simulink library "Scissor_Parts_Lib"  (R2017a)
settings: Solver=ode45  StartTime=0.0  StopTime=10.0  RelTol=1e-3  EnableMultiTasking=on
undefined symbols (not defined in the file): Blue, Extr_Data_LinkHoles, Extr_Data_Ring, Gray, Local, Scissor_Lift_Param, X, Y, Z
libraries: sm_lib x52, Scissor_Parts_Lib x16
(part 1 of 2)
Description:
  | Copyright 2014-2017 The MathWorks, Inc.
settings Model: Creator=smiller  LastModifiedBy=smiller
settings DataIOCC: LimitDataPoints=on  SaveFormat=Array  SignalLoggingSaveFormat=ModelDataLogs
settings OptimizationCC: ExpressionDepthLimit=2147483647  LifeSpan=inf
settings DebuggingCC: UnderspecifiedInitializationDetection=Classic  MergeDetectMultiDrivingBlocksExec=none  SolverPrmCheckMsg=warning  FcnCallInpInsideContextMsg=warning  AllowSymbolicDim=off  StateNameClashWarn=warning  SFUnexpectedBacktrackingDiag=warning  SFNoUnconditionalDefaultTransitionDiag=warning  SFExecutionAtInitializationDiag=none
settings HardwareCC: ProdBitPerPointer=32  ProdBitPerSizeT=32  ProdBitPerPtrDiffT=32  ProdLargestAtomicFloat=None  ProdIntDivRoundTo=Undefined  ProdEndianess=Unspecified  ProdWordSize=32  ProdHWDeviceType=32-bit Generic
settings ModelReferenceCC: PropagateSignalLabelsOutOfModel=off
settings GRTTargetCC: TargetLangStandard=C89/C90 (ANSI)  GeneratePreprocessorConditionals=Disable all
settings ConfigComp: CovMetricSettings=dw  CovHtmlReporting=on  CovSaveCumulativeToWorkspaceVar=on  CovSaveSingleToWorkspaceVar=on  CovExternalEMLEnable=off  CovSFcnEnable=off

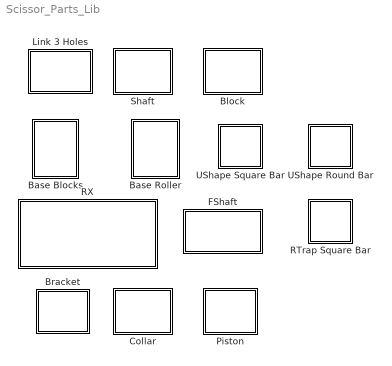
== system Scissor_Parts_Lib ==
  Base Blocks : Subsystem  mask(Base Blocks){block_length=Scissor_Lift_Param.Base_Block.Length, block_width=Scissor_Lift_Param.Base_Block.Width, block_height=Scissor_Lift_Param.Base_Block.Height, shaft_radius=Scissor_Lift_Param.Roller.Shaft_Radius, shaft_length=Scissor_Lift_Param.Roller.Shaft_Length, material_density=Scissor_Lift_Param.Base_Block.Density, material_color=Scissor_Lift_Param.Base_Block.Color, material_opacity=Scissor_Lift_Param.Base_Block.Opacity}
      mask prompts: block_length "Length (cm)"; block_width "Width (cm)"; block_height "Height (cm)"; shaft_radius "Radius (cm)"; shaft_length "Length (cm)"; material_density "Density (kg/m^3)"; material_color "Color"; material_opacity "Opacity"
      mask help: Parameterized base with two blocks and a shaft.
      mask Display:
      | image(imread('Base_Blocks_IMAGE.jpg'));
      | port_label('RConn',1,'S');
      | port_label('LConn',1,'B');
  Base Roller : Subsystem  mask(Base Roller){roller_length=Scissor_Lift_Param.Roller.Roller_Length, roller_radius=Scissor_Lift_Param.Roller.Roller_Radius, shaft_length=Scissor_Lift_Param.Roller.Shaft_Length, shaft_radius=Scissor_Lift_Param.Roller.Shaft_Radius, material_density=Scissor_Lift_Param.Roller.Density, material_color=Scissor_Lift_Param.Roller.Color, material_opacity=Scissor_Lift_Param.Roller.Opacity}
      mask prompts: roller_length "Length (cm)"; roller_radius "Radius (cm)"; shaft_length "Length (cm)"; shaft_radius "Radius (cm)"; material_density "Density (kg/m^3)"; material_color "Color"; material_opacity "Opacity"
      mask help: Parameterized roller with two wheels connected by a shaft.
      mask Display:
      | image(imread('Base_Roller_IMAGE.jpg'));
      | port_label('RConn',1,'S');
      | port_label('LConn',1,'B');
  Block : Subsystem  mask(Block){L=Scissor_Lift_Param.Base_Block.Length, W=Scissor_Lift_Param.Base_Block.Width, H=Scissor_Lift_Param.Base_Block.Height, z_ori=Local +Z, rho=Scissor_Lift_Param.Base_Block.Density, clr=Scissor_Lift_Param.Base_Block.Color, opc=Scissor_Lift_Param.Base_Block.Opacity}
      mask prompts: L "Length (cm):"; W "Width (cm):"; H "Height (cm):"; z_ori "Shaft orientation:"; rho "Shaft density (kg/m^3):"; clr "Link color:"; opc "Opacity:"
      mask help: Rectangular block. Ports are at the center of the faces normal to the local z-axis. Can be configured to have positive Z from B to F or from F to B.
      mask init:
      | if(z_ori == 2)
      |     z_ori = -1;
      | end
      mask TypeOptions z_ori: Local +Z | Local -Z
      mask Display:
      | image(imread('Block_IMAGE.jpg'));
      | port_label('LConn',1,'B');
      | port_label('RConn',1,'F');
  Bracket : Subsystem  mask(Actuation Bracket){fl_w=Scissor_Lift_Param.Actuator.Bracket.Flange.Width, fl_h=Scissor_Lift_Param.Actuator.Bracket.Flange.Height, T=Scissor_Lift_Param.Actuator.Bracket.Flange.Thickness, W=Scissor_Lift_Param.Actuator.Bracket.Flange.Offset, flupdown=Down, flfrontrear=Rear, fl_density=Scissor_Lift_Param.Actuator.Bracket.Flange.Density, fl_clr=Scissor_Lift_Param.Actuator.Bracket.Flange.Color, fl_opc=Scissor_Lift_Param.Actuator.Bracket.Flange.Opacity, shaft_length=Scissor_Lift_Param.Link_Separation.Outer_Outer-Scissor_Lift_Param.Link_Separation.Outer_Inner*2, shaft_radius=Scissor_Lift_Param.Actuator.Bracket.Shaft.Radius, shaft_density=Scissor_Lift_Param.Actuator.Bracket.Shaft.Density, shaft_color=Scissor_Lift_Param.Actuator.Bracket.Shaft.Color, shaft_opacity=Scissor_Lift_Param.Actuator.Bracket.Shaft.Opacity}
      mask prompts: fl_w "Width (cm)"; fl_h "Height (cm)"; T "Thickness (cm)"; W "Offset (cm)"; flupdown "Orientation"; flfrontrear "Position"; fl_density "Density"; fl_clr "Color"; fl_opc "Opacity"; shaft_length "Length (cm)"; shaft_radius "Radius (cm)"; shaft_density "Density (kg/m^3)"; shaft_color "Color"; shaft_opacity "Opacity"
      mask help: Actuation bracket for scissor lift mechanism. Contains flanges that attach to links and connection shaft. Configurable orientation and surface attachment.
      mask init:
      | if(flupdown == 2)
      |     flupdown = -1;
      | end
      | if(flfrontrear == 2)
      |     flfrontrear = -1;
      | end
      mask TypeOptions flupdown: Down | Up
      mask TypeOptions flfrontrear: Front | Rear
      mask Display:
      | image(imread('Bracket_IMAGE.jpg'));
      | port_label('RConn',1,'F');
      | port_label('RConn',2,'B');
      | port_label('LConn',1,'C');
  Collar : Subsystem  mask{collar_length=Scissor_Lift_Param.Actuator.Collar.Length, collar_radius=Scissor_Lift_Param.Actuator.Collar.Radius, cylinder_length=Scissor_Lift_Param.Actuator.Piston_Seat.Length, cylinder_radius=Scissor_Lift_Param.Actuator.Piston_Seat.Radius, cylinder_ori=Local +Z, material_density=Scissor_Lift_Param.Actuator.Collar.Density, material_color=Scissor_Lift_Param.Actuator.Collar.Color, material_opacity=Scissor_Lift_Param.Actuator.Collar.Opacity}
      mask prompts: collar_length "Length (cm):"; collar_radius "Radius (cm):"; cylinder_length "Length (cm):"; cylinder_radius "Radius (cm):"; cylinder_ori "Orientation (B to C):"; material_density "Density (kg/m^3):"; material_color "Color:"; material_opacity "Opacity:"
      mask init:
      | if(cylinder_ori == 2)
      |     cylinder_ori = -1;
      | end
      mask TypeOptions cylinder_ori: Local +Z | Local -Z
      mask Display:
      | image(imread('Actuator_Collar_IMAGE.jpg'));
      | port_label('LConn',1,'B');
      | port_label('RConn',1,'C');
  FShaft : Subsystem  mask(Transverse Shaft){sep_outer_outer=Scissor_Lift_Param.Link_Separation.Outer_Outer, sep_outer_inner=Scissor_Lift_Param.Link_Separation.Outer_Inner, shaft_radius=Scissor_Lift_Param.Trans_Shaft.Radius, shaft_density=Scissor_Lift_Param.Trans_Shaft.Density, shaft_color=Scissor_Lift_Param.Trans_Shaft.Color, shaft_opacity=Scissor_Lift_Param.Trans_Shaft.Opacity}
      mask prompts: sep_outer_outer "Outer connection separation (cm)"; sep_outer_inner "Outer to inner separation (cm)"; shaft_radius "Radius (cm)"; shaft_density "Density (kg/m^3)"; shaft_color "Color"; shaft_opacity "Opacity"
      mask help: Transverse shaft with four connections. Frames are located at shaft center, with Z-axis along center.
      mask Display:
      | image(imread('Shaft_IMAGE.jpg'));
      | port_label('LConn',1,'LO');
      | port_label('LConn',2,'LI');
      | port_label('RConn',1,'RO');
      | port_label('RConn',2,'RI');
  Link 3 Holes : Subsystem  mask(Connector Link, 3 Holes){L=240, W=15, T=4, r=5, rho=1000, clr_string=Gray, opc=1}
      mask prompts: L "Link length (cm):"; W "Link width (cm):"; T "Link thickness (cm):"; r "Hole radius (cm):"; rho "Density (kg/m^3):"; clr_string "Color:"; opc "Opacity:"
      mask help: Connector link with holes. Ports are located at centers of holes, oriented such that Z is out of the hole, positive X is from L hole to R hole.
      mask init:
      | imgfile='Link_3_Hole_Yellow_IMAGE.jpg';
      | if(strcmp(clr_string,'Yellow'))
      |     clr = [0.6 0.6 0.0];
      | elseif(strcmp(clr_string,'Red'))
      |     clr = [0.8 0.2 0.0];
      |     imgfile='Link_3_Hole_Red_IMAGE.jpg';
      | elseif(strcmp(clr_string,'Gray'))
      |     clr = [0.9 0.9 0.9];
      |     imgfile='Link_3_Hole_Gray_IMAGE.jpg';
      | elseif(strcmp(clr_string,'Gray-Blue'))
      |     clr = [164 184 200]/255;
      |     imgfile='Link_3_Hole_GrayBlue_IMAGE.jpg';
      | end
      mask TypeOptions clr_string: Yellow | Red | Gray | Gray-Blue
      mask Display:
      | image(imread(imgfile));
      | port_label('RConn',1,'F');
      | port_label('RConn',2,'C');
      | port_label('RConn',3,'R');
  Piston : Subsystem
      mask Display:
      | image(imread('Piston_Shaft_IMAGE.jpg'));
      | port_label('RConn',1,'P');
      | port_label('LConn',1,'R');
  RTrap Square Bar : Subsystem  mask(U-Shape from Round Bar){pipe_width=5, height_c1=30, height_c2=60, rail_curve_rad1=20, rail_curve_rad2=20, curve_ang1=60, curve_ang2=45, width=150, clr=[0 0.6 0.8], rho=0.01}
      mask prompts: pipe_width "Pipe Width (cm)"; width "Width (cm)"; clr "Color"; rho "Density"
      mask help: U-Shape formed from a bar with square cross-section
      mask DialogControl Control2 Prompt: Curve 1
      mask DialogControl Control3 Prompt: Curve 2
      mask DialogControl Control7 Prompt: Height (cm)
      mask DialogControl Control8 Prompt: Curve Radius (cm)
      mask DialogControl Control9 Prompt: Angle (deg)
  RX : Subsystem  mask(Scissor Lift Crossbar){link_length=Scissor_Lift_Param.Link.Length, link_width=Scissor_Lift_Param.Link.Width, link_thickness=Scissor_Lift_Param.Link.Thickness, link_hole_radius=Scissor_Lift_Param.Link.Hole_Radius, link_density=Scissor_Lift_Param.Link.Density, link_color=Scissor_Lift_Param.Link.Color, link_opacity=Scissor_Lift_Param.Link.Opacity, shaft_length=Scissor_Lift_Param.Link_Separation.Outer_Inner, shaft_radius=Scissor_Lift_Param.Link_Pin.Radius, shaft_density=Scissor_Lift_Param.Link_Pin.Density, shaft_color=Scissor_Lift_Param.Link_Pin.Color, shaft_opacity=Scissor_Lift_Param.Link_Pin.Opacity, leftright=Right, imgfile=Crossbar_RX_IMAGE.jpg, L1Port=OU, L2Port=IU, R1Port=OL, R2Port=IL}
      mask prompts: link_length "Length (cm)"; link_width "Width (cm)"; link_thickness "Thickness (cm)"; link_hole_radius "Hole Radius (cm)"; link_density "Density (kg/m^3)"; link_color "Color"; link_opacity "Opacity"; shaft_length "Length (cm)"; shaft_radius "Radius (cm)"; shaft_density "Density (kg/m^3)"; shaft_color "Color"; shaft_opacity "Opacity"; leftright "Side"; imgfile "Image File"; L1Port "L1 Port Name"; L2Port "L2 Port Name"; R1Port "R1 Port Name"; R2Port "R2 Port Name"
      mask help: Parameterized crossbar. The two links are connected by a revolute joint. Configurable for left or right side.
      mask init:
      | pinbpth = find_system(gcb,'LookUnderMasks','on','FollowLinks','on','Regexp','on','BlockDialogParams','^Local');
      | %get_param(pinbpth,'z_ori')
      | %leftright
      | %if(1==2)
      | if (leftright == 1)
      |     %disp('Setting to 0, LEFT');
      |     set_param(char(pinbpth),'z_ori',1);
      |     set_param([gcb '/OL'],'Port','1','Side','Right');
      |     set_param([gcb '/IL'],'Port','2','Side','Right');
      |     set_param([gcb '/OU'],'Port','3','Side','Left');
      |     set_param([gcb '/IU'],'Port','4','Side','Left');
      |     set_param(gcb,'Name','LX');
      |     L1Port='OU';
      |     L2Port='IU';
      |     R1Port='OL';
      |     R2Port='IL';
      |     imgfile = 'Crossbar_LX_IMAGE.jpg';
      | else
      |     %disp('Setting to 1, RIGHT');
      |     set_param(char(pinbpth),'z_ori',0);
      |     set_param([gcb '/IL'],'Port','1','Side','Right');
      |     set_param([gcb '/OL'],'Port','2','Side','Right');
      |     set_param([gcb '/IU'],'Port','3','Side','Left');
      |     set_param([gcb '/OU'],'Port','4','Side','Left');
      |     set_param(gcb,'Name','RX');
      |     L1Port='IU';
      |     L2Port='OU';
      |     R1Port='IL';
      |     R2Port='OL';
      |     imgfile = 'Crossbar_RX_IMAGE.jpg';
      | end
      | %end
      mask TypeOptions leftright: Left | Right
      mask Display:
      | image(imread(imgfile));
      | port_label('LConn',1,L1Port);
      | port_label('LConn',2,L2Port);
      | port_label('RConn',1,R1Port);
      | port_label('RConn',2,R2Port);
  Shaft : Subsystem  mask(Cylindrical Shaft){L=10, r=5, theta=0, z_ori=Local -Z, Ro=1000, clr=[0.0 0.6 0.8], opc=1}
      mask prompts: L "Length (cm):"; r "Radius (cm):"; theta "Twist (deg)"; z_ori "Orientation (B to F)"; Ro "Density (kg/m^3):"; clr "Color:"; opc "Opacity"
      mask help: Cylindrical shaft. Ports are at shaft ends, and oriented such that the Z-axis is between the ports. Can be configured to have positive Z from B to F or from F to B.
      mask init:
      | if(z_ori == 2)
      |     z_ori = -1;
      | end
      mask TypeOptions z_ori: Local +Z | Local -Z
      mask Display:
      | image(imread('Shaft_IMAGE.jpg'));
      | port_label('LConn',1,'B');
      | port_label('RConn',1,'F');
  UShape Round Bar : Subsystem  mask(U-Shape from Square Bar){pipe_rad=2.5, rail_curve_rad=20, height=150, width=280, clr=[0 0.6 0.8], rho=0.01}
      mask prompts: pipe_rad "Pipe Radius (cm)"; rail_curve_rad "Rail Curve Radius (cm)"; height "Height (cm)"; width "Width (cm)"; clr "Color"; rho "Density"
      mask help: U-Shape formed from a bar with round cross-section
  UShape Square Bar : Subsystem  mask(U-Shape from Round Bar){pipe_width=2.5, rail_curve_rad=20, height=150, width=280, clr=[0 0.6 0.8], rho=0.01}
      mask prompts: pipe_width "Pipe Width (cm)"; rail_curve_rad "Rail Curve Radius (cm)"; height "Height (cm)"; width "Width (cm)"; clr "Color"; rho "Density"
      mask help: U-Shape formed from a bar with square cross-section

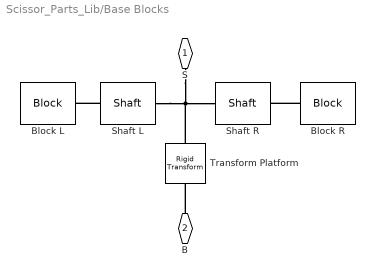
== system Scissor_Parts_Lib/Base Blocks ==
  Block L : Scissor_Parts_Lib/Block  L=block_length  W=block_width  H=block_height  z_ori=Local -Z  rho=material_density  clr=material_color  opc=material_opacity
  Block R : Scissor_Parts_Lib/Block  L=block_length  W=block_width  H=block_height  z_ori=Local +Z  rho=material_density  clr=material_color  opc=material_opacity
  Shaft L : Scissor_Parts_Lib/Shaft  L=shaft_length/2  r=shaft_radius  theta=0  z_ori=Local -Z  Ro=material_density  clr=material_color  opc=material_opacity
  Shaft R : Scissor_Parts_Lib/Shaft  L=shaft_length/2  r=shaft_radius  theta=0  z_ori=Local +Z  Ro=material_density  clr=material_color  opc=material_opacity
  Transform Platform : sm_lib/Frames and Transforms/Rigid Transform  TranslationMethod=Cartesian  TranslationStandardOffset=Scissor_Lift_Param.Roller.Roller_Radius  TranslationLengthUnit=cm  TranslationStandardAxis=-Y  TranslationCartesianOffset=[0 -block_height/2 0]  TranslationROffset=0  TranslationROffsetUnits=m  TranslationZOffset=0  TranslationZOffsetUnits=m  TranslationThetaOffset=0  TranslationThetaOffsetUnits=deg  RotationMethod=None  RotationAngleUnits=deg  RotationStandardAxis=+Y  RotationAngle=0  RotationArbitraryAxis=[0 0 1]  FollAlignAxisA=+X  BaseAlignAxisA=+Y  FollAlignAxisB=+Y  BaseAlignAxisB=+Z  RotationSequenceAxes=FollowerAxes  RotationSequence=XYX  RotationSequenceAngles=[0 0 0]  RotationSequenceAnglesUnits=deg  RotationMatrix=[1 0 0; 0 1 0; 0 0 1]
  S : PMIOPort  Port=1  Side=Right
  B : PMIOPort  Port=2  Side=Left
  connections:
  Shaft L/RConn1 -- Block L/LConn1
  Block R/LConn1 -- Shaft R/RConn1
  B/RConn1 -- Transform Platform/RConn1
  Shaft L/LConn1 -- Shaft R/LConn1 -- Transform Platform/LConn1 -- S/RConn1

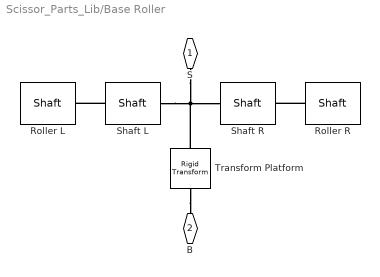
== system Scissor_Parts_Lib/Base Roller ==
  Roller L : Scissor_Parts_Lib/Shaft  L=roller_length  r=roller_radius  theta=0  z_ori=Local -Z  Ro=material_density  clr=material_color  opc=material_opacity
  Roller R : Scissor_Parts_Lib/Shaft  L=roller_length  r=roller_radius  theta=0  z_ori=Local +Z  Ro=material_density  clr=material_color  opc=material_opacity
  Shaft L : Scissor_Parts_Lib/Shaft  L=shaft_length/2  r=shaft_radius  theta=0  z_ori=Local -Z  Ro=material_density  clr=material_color  opc=material_opacity
  Shaft R : Scissor_Parts_Lib/Shaft  L=shaft_length/2  r=shaft_radius  theta=0  z_ori=Local +Z  Ro=material_density  clr=material_color  opc=material_opacity
  Transform Platform : sm_lib/Frames and Transforms/Rigid Transform  TranslationMethod=None  TranslationStandardOffset=0  TranslationLengthUnit=cm  TranslationStandardAxis=-Y  TranslationCartesianOffset=[0 0 0]  TranslationROffset=0  TranslationROffsetUnits=m  TranslationZOffset=0  TranslationZOffsetUnits=m  TranslationThetaOffset=0  TranslationThetaOffsetUnits=deg  RotationMethod=StandardAxis  RotationAngleUnits=deg  RotationStandardAxis=+Y  RotationAngle=90  RotationArbitraryAxis=[0 0 1]  FollAlignAxisA=+X  BaseAlignAxisA=+Y  FollAlignAxisB=+Y  BaseAlignAxisB=+Z  RotationSequenceAxes=FollowerAxes  RotationSequence=XYX  RotationSequenceAngles=[0 0 0]  RotationSequenceAnglesUnits=deg  RotationMatrix=[1 0 0; 0 1 0; 0 0 1]
  S : PMIOPort  Port=1  Side=Right
  B : PMIOPort  Port=2  Side=Left
  connections:
  Shaft L/RConn1 -- Roller L/LConn1
  Roller R/LConn1 -- Shaft R/RConn1
  S/RConn1 -- Transform Platform/LConn1 -- Shaft L/LConn1 -- Shaft R/LConn1
  Transform Platform/RConn1 -- B/RConn1

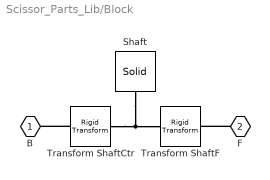
== system Scissor_Parts_Lib/Block ==
  Shaft : sm_lib/Body Elements/Solid  InertiaType=CalculateFromGeometry  Mass=1  MassUnits=kg  CenterOfMass=[0 0 0]  CenterOfMassUnits=m  MomentsOfInertia=[1 1 1]  MomentsOfInertiaUnits=kg*m^2  ProductsOfInertia=[0 0 0]  ProductsOfInertiaUnits=kg*m^2  DensityBased=on  Density=rho  DensityUnits=kg/m^3  DoExposeReferenceFrame=on  SerializedFrames=<Frames/>  GraphicType=FromGeometry  MarkerShape=Sphere  MarkerSize=1  MarkerSizeUnits=m  GraphicVisPropType=SimpleVisualProperties  GraphicDiffuseColor=clr  GraphicSpecularColor=[0.2 0.2 0.2]  GraphicAmbientColor=[0.5 0.5 0.5]  GraphicEmissiveColor=[0.1 0.1 0.1]  GraphicShininess=24.0  GraphicOpacity=opc  GeometryShape=Brick  RectangleSize=[1 1]  RectangleSizeUnits=m  BrickDimensions=[W H L]  BrickDimensionUnits=cm  CylinderRadius=1  CylinderRadiusUnits=cm  CylinderLength=1  CylinderLengthUnits=cm  SphereRadius=1  SphereRadiusUnits=m  EllipsoidRadii=[1 1 1]  EllipsoidRadiiUnits=m  ExtrusionCrossSection=[1 1; -1 1; -1 -1; 1 -1]  ExtrusionCrossSectionUnits=m  ExtrusionLength=1  ExtrusionLengthUnits=m  PolygonNumSides=1  PolygonOuterRadius=1  PolygonOuterRadiusUnits=m  ExtGeomFileType=STEP  ExtGeomFileUnits=m  RevolutionCrossSection=[1 1; 1 -1; 2 -1; 2 1]  RevolutionCrossSectionUnits=m  RevolutionExtent=Full  RevolutionAngle=180  RevolutionAngleUnits=deg
  Transform ShaftCtr : sm_lib/Frames and Transforms/Rigid Transform  TranslationMethod=Cartesian  TranslationStandardOffset=0  TranslationLengthUnit=cm  TranslationStandardAxis=+Z  TranslationCartesianOffset=[0 0 L/2]*z_ori  TranslationROffset=0  TranslationROffsetUnits=m  TranslationZOffset=0  TranslationZOffsetUnits=m  TranslationThetaOffset=0  TranslationThetaOffsetUnits=deg  RotationMethod=None  RotationAngleUnits=deg  RotationStandardAxis=+Z  RotationAngle=0  RotationArbitraryAxis=[0 0 1]  FollAlignAxisA=+X  BaseAlignAxisA=+Y  FollAlignAxisB=+Y  BaseAlignAxisB=+Z  RotationSequenceAxes=FollowerAxes  RotationSequence=XYX  RotationSequenceAngles=[0 0 0]  RotationSequenceAnglesUnits=deg  RotationMatrix=[1 0 0; 0 1 0; 0 0 1]
  Transform ShaftF : sm_lib/Frames and Transforms/Rigid Transform  TranslationMethod=Cartesian  TranslationStandardOffset=0  TranslationLengthUnit=cm  TranslationStandardAxis=+Z  TranslationCartesianOffset=[0 0 L/2]*z_ori  TranslationROffset=0  TranslationROffsetUnits=m  TranslationZOffset=0  TranslationZOffsetUnits=m  TranslationThetaOffset=0  TranslationThetaOffsetUnits=deg  RotationMethod=None  RotationAngleUnits=deg  RotationStandardAxis=+Z  RotationAngle=0  RotationArbitraryAxis=[0 0 1]  FollAlignAxisA=+X  BaseAlignAxisA=+Y  FollAlignAxisB=+Y  BaseAlignAxisB=+Z  RotationSequenceAxes=FollowerAxes  RotationSequence=XYX  RotationSequenceAngles=[0 0 0]  RotationSequenceAnglesUnits=deg  RotationMatrix=[1 0 0; 0 1 0; 0 0 1]
  B : PMIOPort  Port=1  Side=Left
  F : PMIOPort  Port=2  Side=Right
  connections:
  Transform ShaftCtr/LConn1 -- B/RConn1
  F/RConn1 -- Transform ShaftF/RConn1
  Shaft/RConn1 -- Transform ShaftF/LConn1 -- Transform ShaftCtr/RConn1

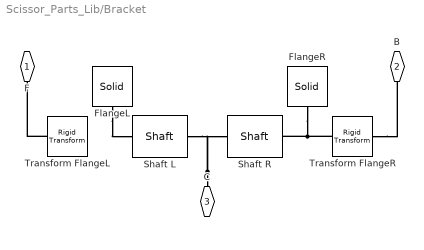
== system Scissor_Parts_Lib/Bracket ==
  FlangeL : sm_lib/Body Elements/Solid  InertiaType=CalculateFromGeometry  Mass=1  MassUnits=kg  CenterOfMass=[0 0 0]  CenterOfMassUnits=m  MomentsOfInertia=[1 1 1]  MomentsOfInertiaUnits=kg*m^2  ProductsOfInertia=[0 0 0]  ProductsOfInertiaUnits=kg*m^2  DensityBased=on  Density=fl_density  DensityUnits=kg/m^3  DoExposeReferenceFrame=on  SerializedFrames=<Frames/>  GraphicType=FromGeometry  MarkerShape=Sphere  MarkerSize=1  MarkerSizeUnits=m  GraphicVisPropType=SimpleVisualProperties  GraphicDiffuseColor=fl_clr  GraphicSpecularColor=[0.2 0.2 0.2]  GraphicAmbientColor=[0.5 0.5 0.5]  GraphicEmissiveColor=[0.1 0.1 0.1]  GraphicShininess=24.0  GraphicOpacity=fl_opc  GeometryShape=GeneralExtrusion  RectangleSize=[1 1]  RectangleSizeUnits=m  BrickDimensions=[1 1 1]  BrickDimensionUnits=m  CylinderRadius=1  CylinderRadiusUnits=m  CylinderLength=1  CylinderLengthUnits=m  SphereRadius=1  SphereRadiusUnits=m  EllipsoidRadii=[1 1 1]  EllipsoidRadiiUnits=m  ExtrusionCrossSection=[0 fl_h;-fl_w -fl_h;fl_w -fl_h]*0.5*flupdown  ExtrusionCrossSectionUnits=cm  ExtrusionLength=T  ExtrusionLengthUnits=cm  PolygonNumSides=1  PolygonOuterRadius=1  PolygonOuterRadiusUnits=m  ExtGeomFileType=STEP  ExtGeomFileUnits=m  RevolutionCrossSection=[1 1; 1 -1; 2 -1; 2 1]  RevolutionCrossSectionUnits=m  RevolutionExtent=Full  RevolutionAngle=180  RevolutionAngleUnits=deg
  FlangeR : sm_lib/Body Elements/Solid  InertiaType=CalculateFromGeometry  Mass=1  MassUnits=kg  CenterOfMass=[0 0 0]  CenterOfMassUnits=m  MomentsOfInertia=[1 1 1]  MomentsOfInertiaUnits=kg*m^2  ProductsOfInertia=[0 0 0]  ProductsOfInertiaUnits=kg*m^2  DensityBased=on  Density=fl_density  DensityUnits=kg/m^3  DoExposeReferenceFrame=on  SerializedFrames=<Frames/>  GraphicType=FromGeometry  MarkerShape=Sphere  MarkerSize=1  MarkerSizeUnits=m  GraphicVisPropType=SimpleVisualProperties  GraphicDiffuseColor=fl_clr  GraphicSpecularColor=[0.2 0.2 0.2]  GraphicAmbientColor=[0.5 0.5 0.5]  GraphicEmissiveColor=[0.1 0.1 0.1]  GraphicShininess=24.0  GraphicOpacity=fl_opc  GeometryShape=GeneralExtrusion  RectangleSize=[1 1]  RectangleSizeUnits=m  BrickDimensions=[1 1 1]  BrickDimensionUnits=m  CylinderRadius=1  CylinderRadiusUnits=m  CylinderLength=1  CylinderLengthUnits=m  SphereRadius=1  SphereRadiusUnits=m  EllipsoidRadii=[1 1 1]  EllipsoidRadiiUnits=m  ExtrusionCrossSection=[0 fl_h;-fl_w -fl_h;fl_w -fl_h]*0.5*flupdown  ExtrusionCrossSectionUnits=cm  ExtrusionLength=T  ExtrusionLengthUnits=cm  PolygonNumSides=1  PolygonOuterRadius=1  PolygonOuterRadiusUnits=m  ExtGeomFileType=STEP  ExtGeomFileUnits=m  RevolutionCrossSection=[1 1; 1 -1; 2 -1; 2 1]  RevolutionCrossSectionUnits=m  RevolutionExtent=Full  RevolutionAngle=180  RevolutionAngleUnits=deg
  Shaft L : Scissor_Parts_Lib/Shaft  L=shaft_length/2  r=shaft_radius  theta=0  z_ori=Local -Z  Ro=shaft_density  clr=shaft_color  opc=shaft_opacity
  Shaft R : Scissor_Parts_Lib/Shaft  L=shaft_length/2  r=shaft_radius  theta=0  z_ori=Local -Z  Ro=shaft_density  clr=shaft_color  opc=shaft_opacity
  Transform FlangeL : sm_lib/Frames and Transforms/Rigid Transform  TranslationMethod=Cartesian  TranslationStandardOffset=1  TranslationLengthUnit=cm  TranslationStandardAxis=-X  TranslationCartesianOffset=[(fl_w/2)*flfrontrear (fl_h/2+W/2)*flupdown 0]  TranslationROffset=0  TranslationROffsetUnits=m  TranslationZOffset=0  TranslationZOffsetUnits=m  TranslationThetaOffset=0  TranslationThetaOffsetUnits=deg  RotationMethod=None  RotationAngleUnits=deg  RotationStandardAxis=+Z  RotationAngle=0  RotationArbitraryAxis=[0 0 1]  FollAlignAxisA=+X  BaseAlignAxisA=+Y  FollAlignAxisB=+Y  BaseAlignAxisB=+Z  RotationSequenceAxes=FollowerAxes  RotationSequence=XYX  RotationSequenceAngles=[0 0 0]  RotationSequenceAnglesUnits=deg  RotationMatrix=[1 0 0; 0 1 0; 0 0 1]
  Transform FlangeR : sm_lib/Frames and Transforms/Rigid Transform  TranslationMethod=Cartesian  TranslationStandardOffset=1  TranslationLengthUnit=cm  TranslationStandardAxis=-X  TranslationCartesianOffset=[(fl_w/2)*flfrontrear (fl_h/2+W/2)*flupdown 0]  TranslationROffset=0  TranslationROffsetUnits=m  TranslationZOffset=0  TranslationZOffsetUnits=m  TranslationThetaOffset=0  TranslationThetaOffsetUnits=deg  RotationMethod=None  RotationAngleUnits=deg  RotationStandardAxis=+Z  RotationAngle=0  RotationArbitraryAxis=[0 0 1]  FollAlignAxisA=+X  BaseAlignAxisA=+Y  FollAlignAxisB=+Y  BaseAlignAxisB=+Z  RotationSequenceAxes=FollowerAxes  RotationSequence=XYX  RotationSequenceAngles=[0 0 0]  RotationSequenceAnglesUnits=deg  RotationMatrix=[1 0 0; 0 1 0; 0 0 1]
  F : PMIOPort  Port=1  Side=Right
  B : PMIOPort  Port=2  Side=Right
  C : PMIOPort  Port=3  Side=Left
  connections:
  Transform FlangeL/LConn1 -- F/RConn1
  Transform FlangeR/LConn1 -- B/RConn1
  FlangeR/RConn1 -- Shaft R/RConn1 -- Transform FlangeR/RConn1
  FlangeL/RConn1 -- Shaft L/LConn1
  C/RConn1 -- Shaft L/RConn1 -- Shaft R/LConn1

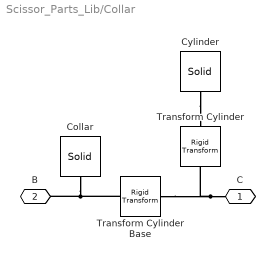
== system Scissor_Parts_Lib/Collar ==
  Collar : sm_lib/Body Elements/Solid  InertiaType=CalculateFromGeometry  Mass=1  MassUnits=kg  CenterOfMass=[0 0 0]  CenterOfMassUnits=m  MomentsOfInertia=[1 1 1]  MomentsOfInertiaUnits=kg*m^2  ProductsOfInertia=[0 0 0]  ProductsOfInertiaUnits=kg*m^2  DensityBased=on  Density=material_density  DensityUnits=kg/(m^3)  DoExposeReferenceFrame=on  SerializedFrames=<Frames/>  GraphicType=FromGeometry  MarkerShape=Sphere  MarkerSize=10  MarkerSizeUnits=m  GraphicVisPropType=SimpleVisualProperties  GraphicDiffuseColor=material_color  GraphicSpecularColor=[0.5 0.5 0.5 1.0]  GraphicAmbientColor=[0.15 0.15 0.15 1.0]  GraphicEmissiveColor=[0.0 0.0 0.0 1.0]  GraphicShininess=75  GraphicOpacity=material_opacity  GeometryShape=GeneralExtrusion  RectangleSize=[1 1]  RectangleSizeUnits=m  BrickDimensions=[10 10 100]  BrickDimensionUnits=cm  CylinderRadius=Scissor_Lift_Param.Trans_Shaft.Radius*1.3  CylinderRadiusUnits=cm  CylinderLength=1  CylinderLengthUnits=cm  SphereRadius=1  SphereRadiusUnits=m  EllipsoidRadii=[1 1 1]  EllipsoidRadiiUnits=m  ExtrusionCrossSection=Extr_Data_Ring(collar_radius,collar_radius*0.9,0,360)  ExtrusionCrossSectionUnits=cm  ExtrusionLength=collar_length  ExtrusionLengthUnits=cm  PolygonNumSides=3  PolygonOuterRadius=1  PolygonOuterRadiusUnits=m  ExtGeomFileType=STL  ExtGeomFileUnits=m  RevolutionCrossSection=[1 1; 1 -1; 2 -1; 2 1]  RevolutionCrossSectionUnits=m  RevolutionExtent=Full  RevolutionAngle=180  RevolutionAngleUnits=deg
  Cylinder : sm_lib/Body Elements/Solid  InertiaType=CalculateFromGeometry  Mass=1  MassUnits=kg  CenterOfMass=[0 0 0]  CenterOfMassUnits=m  MomentsOfInertia=[1 1 1]  MomentsOfInertiaUnits=kg*m^2  ProductsOfInertia=[0 0 0]  ProductsOfInertiaUnits=kg*m^2  DensityBased=on  Density=material_density  DensityUnits=kg/(m^3)  DoExposeReferenceFrame=on  SerializedFrames=<Frames/>  GraphicType=FromGeometry  MarkerShape=Sphere  MarkerSize=10  MarkerSizeUnits=m  GraphicVisPropType=SimpleVisualProperties  GraphicDiffuseColor=material_color  GraphicSpecularColor=[0.5 0.5 0.5 1.0]  GraphicAmbientColor=[0.15 0.15 0.15 1.0]  GraphicEmissiveColor=[0.0 0.0 0.0 1.0]  GraphicShininess=75  GraphicOpacity=material_opacity  GeometryShape=GeneralExtrusion  RectangleSize=[1 1]  RectangleSizeUnits=m  BrickDimensions=[10 10 100]  BrickDimensionUnits=cm  CylinderRadius=Scissor_Lift_Param.Trans_Shaft.Radius*1.3  CylinderRadiusUnits=cm  CylinderLength=1  CylinderLengthUnits=cm  SphereRadius=1  SphereRadiusUnits=m  EllipsoidRadii=[1 1 1]  EllipsoidRadiiUnits=m  ExtrusionCrossSection=Extr_Data_Ring(cylinder_radius,cylinder_radius*0.9,0,360)  ExtrusionCrossSectionUnits=cm  ExtrusionLength=cylinder_length  ExtrusionLengthUnits=cm  PolygonNumSides=3  PolygonOuterRadius=1  PolygonOuterRadiusUnits=m  ExtGeomFileType=STEP  ExtGeomFileUnits=m  RevolutionCrossSection=[1 1; 1 -1; 2 -1; 2 1]  RevolutionCrossSectionUnits=m  RevolutionExtent=Full  RevolutionAngle=180  RevolutionAngleUnits=deg
  Transform Cylinder : sm_lib/Frames and Transforms/Rigid Transform  TranslationMethod=StandardAxis  TranslationStandardOffset=cylinder_length/2*cylinder_ori  TranslationLengthUnit=cm  TranslationStandardAxis=+Z  TranslationCartesianOffset=[0 0 0]  TranslationROffset=0  TranslationROffsetUnits=m  TranslationZOffset=0  TranslationZOffsetUnits=m  TranslationThetaOffset=0  TranslationThetaOffsetUnits=deg  RotationMethod=None  RotationAngleUnits=deg  RotationStandardAxis=+Y  RotationAngle=0  RotationArbitraryAxis=[0 0 1]  FollAlignAxisA=+X  BaseAlignAxisA=+Y  FollAlignAxisB=+Y  BaseAlignAxisB=+Z  RotationSequenceAxes=FollowerAxes  RotationSequence=XYX  RotationSequenceAngles=[0 0 0]  RotationSequenceAnglesUnits=deg  RotationMatrix=[1 0 0; 0 1 0; 0 0 1]
  Transform Cylinder Base : sm_lib/Frames and Transforms/Rigid Transform  TranslationMethod=None  TranslationStandardOffset=0  TranslationLengthUnit=m  TranslationStandardAxis=+Z  TranslationCartesianOffset=[0 0 0]  TranslationROffset=0  TranslationROffsetUnits=m  TranslationZOffset=0  TranslationZOffsetUnits=m  TranslationThetaOffset=0  TranslationThetaOffsetUnits=deg  RotationMethod=StandardAxis  RotationAngleUnits=deg  RotationStandardAxis=-Y  RotationAngle=90  RotationArbitraryAxis=[0 0 1]  FollAlignAxisA=+X  BaseAlignAxisA=+Y  FollAlignAxisB=+Y  BaseAlignAxisB=+Z  RotationSequenceAxes=FollowerAxes  RotationSequence=XYX  RotationSequenceAngles=[0 0 0]  RotationSequenceAnglesUnits=deg  RotationMatrix=[1 0 0; 0 1 0; 0 0 1]
  C : PMIOPort  Port=1  Side=Right
  B : PMIOPort  Port=2  Side=Left
  connections:
  Transform Cylinder Base/LConn1 -- Collar/RConn1 -- B/RConn1
  Cylinder/RConn1 -- Transform Cylinder/RConn1
  C/RConn1 -- Transform Cylinder Base/RConn1 -- Transform Cylinder/LConn1

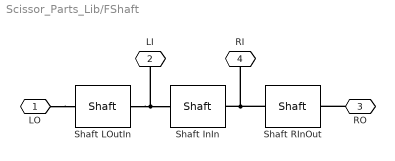
== system Scissor_Parts_Lib/FShaft ==
  Shaft InIn : Scissor_Parts_Lib/Shaft  L=sep_outer_outer-2*sep_outer_inner  r=shaft_radius  theta=0  z_ori=Local -Z  Ro=shaft_density  clr=shaft_color  opc=shaft_opacity
  Shaft LOutIn : Scissor_Parts_Lib/Shaft  L=sep_outer_inner  r=shaft_radius  theta=0  z_ori=Local -Z  Ro=shaft_density  clr=shaft_color  opc=shaft_opacity
  Shaft RInOut : Scissor_Parts_Lib/Shaft  L=sep_outer_inner  r=shaft_radius  theta=0  z_ori=Local -Z  Ro=shaft_density  clr=shaft_color  opc=shaft_opacity
  LO : PMIOPort  Port=1  Side=Left
  LI : PMIOPort  Port=2  Side=Left
  RO : PMIOPort  Port=3  Side=Right
  RI : PMIOPort  Port=4  Side=Right
  connections:
  Shaft LOutIn/RConn1 -- LI/RConn1 -- Shaft InIn/LConn1
  Shaft RInOut/LConn1 -- Shaft InIn/RConn1 -- RI/RConn1
  LO/RConn1 -- Shaft LOutIn/LConn1
  RO/RConn1 -- Shaft RInOut/RConn1

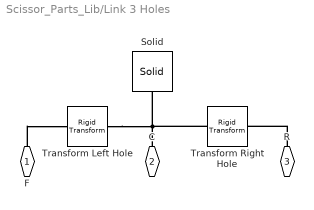
== system Scissor_Parts_Lib/Link 3 Holes ==
  Solid : sm_lib/Body Elements/Solid  InertiaType=CalculateFromGeometry  Mass=1  MassUnits=kg  CenterOfMass=[0 0 0]  CenterOfMassUnits=m  MomentsOfInertia=[1 1 1]  MomentsOfInertiaUnits=kg*m^2  ProductsOfInertia=[0 0 0]  ProductsOfInertiaUnits=kg*m^2  DensityBased=on  Density=rho  DensityUnits=kg/(m^3)  DoExposeReferenceFrame=on  SerializedFrames=<Frames/>  GraphicType=FromGeometry  MarkerShape=Sphere  MarkerSize=10  GraphicVisPropType=SimpleVisualProperties  GraphicDiffuseColor=clr  GraphicSpecularColor=[0.5 0.5 0.5 1.0]  GraphicAmbientColor=[0.15 0.15 0.15 1.0]  GraphicEmissiveColor=[0.0 0.0 0.0 1.0]  GraphicShininess=75  GraphicOpacity=opc  GeometryShape=GeneralExtrusion  RectangleSize=[1 1]  RectangleSizeUnits=m  BrickDimensions=[1 1 1]*0.01  BrickDimensionUnits=m  CylinderRadius=1  CylinderRadiusUnits=m  CylinderLength=1  CylinderLengthUnits=m  SphereRadius=1  SphereRadiusUnits=m  EllipsoidRadii=[1 1 1]  EllipsoidRadiiUnits=m  ExtrusionCrossSection=Extr_Data_LinkHoles(L,W,r,3)  ExtrusionCrossSectionUnits=cm  ExtrusionLength=T  ExtrusionLengthUnits=cm  PolygonNumSides=3  PolygonOuterRadius=1  PolygonOuterRadiusUnits=m  ExtGeomFileType=STEP  ExtGeomFileUnits=m  RevolutionCrossSection=[1 1; 1 -1; 2 -1; 2 1]  RevolutionCrossSectionUnits=m  RevolutionExtent=Full  RevolutionAngle=180  RevolutionAngleUnits=deg
  Transform Left Hole : sm_lib/Frames and Transforms/Rigid Transform  TranslationMethod=StandardAxis  TranslationStandardOffset=L/2  TranslationLengthUnit=cm  TranslationStandardAxis=+X  TranslationCartesianOffset=[0 0 0]  TranslationROffset=0  TranslationROffsetUnits=m  TranslationZOffset=0  TranslationZOffsetUnits=m  TranslationThetaOffset=0  TranslationThetaOffsetUnits=deg  RotationMethod=None  RotationAngleUnits=deg  RotationStandardAxis=+Z  RotationAngle=0  RotationArbitraryAxis=[0 0 1]  FollAlignAxisA=+X  BaseAlignAxisA=+Y  FollAlignAxisB=+Y  BaseAlignAxisB=+Z  RotationSequenceAxes=FollowerAxes  RotationSequence=XYX  RotationSequenceAngles=[0 0 0]  RotationSequenceAnglesUnits=deg  RotationMatrix=[1 0 0; 0 1 0; 0 0 1]
  Transform Right Hole : sm_lib/Frames and Transforms/Rigid Transform  TranslationMethod=StandardAxis  TranslationStandardOffset=L/2  TranslationLengthUnit=cm  TranslationStandardAxis=+X  TranslationCartesianOffset=[0 0 0]  TranslationROffset=0  TranslationROffsetUnits=m  TranslationZOffset=0  TranslationZOffsetUnits=m  TranslationThetaOffset=0  TranslationThetaOffsetUnits=deg  RotationMethod=None  RotationAngleUnits=deg  RotationStandardAxis=+Z  RotationAngle=0  RotationArbitraryAxis=[0 0 1]  FollAlignAxisA=+X  BaseAlignAxisA=+Y  FollAlignAxisB=+Y  BaseAlignAxisB=+Z  RotationSequenceAxes=FollowerAxes  RotationSequence=XYX  RotationSequenceAngles=[0 0 0]  RotationSequenceAnglesUnits=deg  RotationMatrix=[1 0 0; 0 1 0; 0 0 1]
  F : PMIOPort  Port=1  Side=Right
  C : PMIOPort  Port=2  Side=Right
  R : PMIOPort  Port=3  Side=Right
  connections:
  Transform Left Hole/RConn1 -- Transform Right Hole/LConn1 -- Solid/RConn1 -- C/RConn1
  R/RConn1 -- Transform Right Hole/RConn1
  F/RConn1 -- Transform Left Hole/LConn1

== system Scissor_Parts_Lib/Piston ==
  Piston : sm_lib/Body Elements/Solid  InertiaType=CalculateFromGeometry  Mass=1  MassUnits=kg  CenterOfMass=[0 0 0]  CenterOfMassUnits=m  MomentsOfInertia=[1 1 1]  MomentsOfInertiaUnits=kg*m^2  ProductsOfInertia=[0 0 0]  ProductsOfInertiaUnits=kg*m^2  DensityBased=on  Density=1000  DensityUnits=kg/(m^3)  DoExposeReferenceFrame=on  SerializedFrames=<Frames/>  GraphicType=FromGeometry  MarkerShape=Sphere  MarkerSize=10  MarkerSizeUnits=m  GraphicVisPropType=SimpleVisualProperties  GraphicDiffuseColor=[0.8 0.8 0.8]  GraphicSpecularColor=[0.5 0.5 0.5 1.0]  GraphicAmbientColor=[0.15 0.15 0.15 1.0]  GraphicEmissiveColor=[0.0 0.0 0.0 1.0]  GraphicShininess=75  GraphicOpacity=1.0  GeometryShape=Cylinder  RectangleSize=[1 1]  RectangleSizeUnits=m  BrickDimensions=[10 10 100]  BrickDimensionUnits=cm  CylinderRadius=Scissor_Lift_Param.Actuator.Piston_Radius  CylinderRadiusUnits=cm  CylinderLength=Scissor_Lift_Param.Actuator.Piston_Length  CylinderLengthUnits=cm  SphereRadius=1  SphereRadiusUnits=m  EllipsoidRadii=[1 1 1]  EllipsoidRadiiUnits=m  ExtrusionCrossSection=[1 1;1 -1;-1 -1;-1 1]  ExtrusionCrossSectionUnits=cm  ExtrusionLength=1  ExtrusionLengthUnits=cm  PolygonNumSides=3  PolygonOuterRadius=1  PolygonOuterRadiusUnits=m  ExtGeomFileType=STEP  ExtGeomFileUnits=m  RevolutionCrossSection=[1 1; 1 -1; 2 -1; 2 1]  RevolutionCrossSectionUnits=m  RevolutionExtent=Full  RevolutionAngle=180  RevolutionAngleUnits=deg
  Transform Piston CG : sm_lib/Frames and Transforms/Rigid Transform  TranslationMethod=StandardAxis  TranslationStandardOffset=Scissor_Lift_Param.Actuator.Piston_Length/2  TranslationLengthUnit=cm  TranslationStandardAxis=-Z  TranslationCartesianOffset=[0 0 0]  TranslationROffset=0  TranslationROffsetUnits=m  TranslationZOffset=0  TranslationZOffsetUnits=m  TranslationThetaOffset=0  TranslationThetaOffsetUnits=deg  RotationMethod=None  RotationAngleUnits=deg  RotationStandardAxis=+Y  RotationAngle=0  RotationArbitraryAxis=[0 0 1]  FollAlignAxisA=+X  BaseAlignAxisA=+Y  FollAlignAxisB=+Y  BaseAlignAxisB=+Z  RotationSequenceAxes=FollowerAxes  RotationSequence=XYX  RotationSequenceAngles=[0 0 0]  RotationSequenceAnglesUnits=deg  RotationMatrix=[1 0 0; 0 1 0; 0 0 1]
  C : PMIOPort  Port=1  Side=Left
  P : PMIOPort  Port=2  Side=Right
  connections:
  Piston/RConn1 -- Transform Piston CG/RConn1
  C/RConn1 -- Transform Piston CG/LConn1 -- P/RConn1

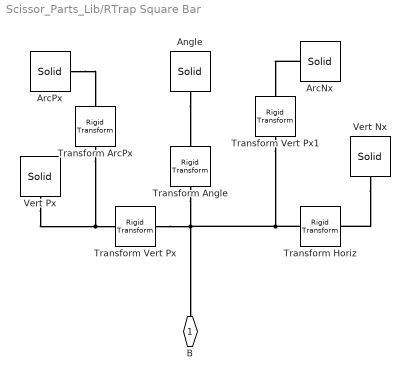
== system Scissor_Parts_Lib/RTrap Square Bar ==
  Angle : sm_lib/Body Elements/Solid  InertiaType=CalculateFromGeometry  Mass=1  MassUnits=kg  CenterOfMass=[0 0 0]  CenterOfMassUnits=m  MomentsOfInertia=[1 1 1]  MomentsOfInertiaUnits=kg*m^2  ProductsOfInertia=[0 0 0]  ProductsOfInertiaUnits=kg*m^2  DensityBased=on  Density=rho  DensityUnits=kg/(m^3)  DoExposeReferenceFrame=on  SerializedFrames=<Frames/>  GraphicType=FromGeometry  MarkerShape=Sphere  MarkerSize=10  GraphicVisPropType=SimpleVisualProperties  GraphicDiffuseColor=clr  GraphicSpecularColor=[0.5 0.5 0.5 1.0]  GraphicAmbientColor=[0.15 0.15 0.15 1.0]  GraphicEmissiveColor=[0.0 0.0 0.0 1.0]  GraphicShininess=75  GraphicOpacity=1.0  GeometryShape=Brick  RectangleSize=[1 1]  RectangleSizeUnits=m  BrickDimensions=[pipe_width pipe_width (height_c2-height_c1)/sind(90-curve_ang1)]  BrickDimensionUnits=cm  CylinderRadius=1  CylinderRadiusUnits=cm  CylinderLength=1  CylinderLengthUnits=cm  SphereRadius=1  SphereRadiusUnits=m  EllipsoidRadii=[1 1 1]  EllipsoidRadiiUnits=m  ExtrusionCrossSection=[1 1; -1 1; -1 -1; 1 -1]  ExtrusionCrossSectionUnits=m  ExtrusionLength=1  ExtrusionLengthUnits=m  PolygonNumSides=3  PolygonOuterRadius=1  PolygonOuterRadiusUnits=m  ExtGeomFileType=STEP  ExtGeomFileUnits=m  RevolutionCrossSection=[1 1; 1 -1; 2 -1; 2 1]  RevolutionCrossSectionUnits=m  RevolutionExtent=Full  RevolutionAngle=180  RevolutionAngleUnits=deg
  ArcNx : sm_lib/Body Elements/Solid  InertiaType=CalculateFromGeometry  Mass=1  MassUnits=kg  CenterOfMass=[0 0 0]  CenterOfMassUnits=m  MomentsOfInertia=[1 1 1]  MomentsOfInertiaUnits=kg*m^2  ProductsOfInertia=[0 0 0]  ProductsOfInertiaUnits=kg*m^2  DensityBased=on  Density=rho  DensityUnits=kg/(m^3)  DoExposeReferenceFrame=on  SerializedFrames=<Frames/>  GraphicType=FromGeometry  MarkerShape=Sphere  MarkerSize=10  GraphicVisPropType=SimpleVisualProperties  GraphicDiffuseColor=clr  GraphicSpecularColor=[0.5 0.5 0.5 1.0]  GraphicAmbientColor=[0.15 0.15 0.15 1.0]  GraphicEmissiveColor=[0.0 0.0 0.0 1.0]  GraphicShininess=75  GraphicOpacity=1.0  GeometryShape=GeneralSolidOfRevolution  RectangleSize=[1 1]  RectangleSizeUnits=m  BrickDimensions=[1 1 1]  BrickDimensionUnits=m  CylinderRadius=1  CylinderRadiusUnits=m  CylinderLength=1  CylinderLengthUnits=m  SphereRadius=1  SphereRadiusUnits=m  EllipsoidRadii=[1 1 1]  EllipsoidRadiiUnits=m  ExtrusionCrossSection=[1 1; -1 1; -1 -1; 1 -1]  ExtrusionCrossSectionUnits=m  ExtrusionLength=1  ExtrusionLengthUnits=m  PolygonNumSides=3  PolygonOuterRadius=1  PolygonOuterRadiusUnits=m  ExtGeomFileType=STEP  ExtGeomFileUnits=m  RevolutionCrossSection=[[-1 1 1 -1]*pipe_width/2+rail_curve_rad1;[-1 -1 1 1]*pipe_width/2]'  RevolutionCrossSectionUnits=cm  RevolutionExtent=Custom  RevolutionAngle=90-curve_ang1  RevolutionAngleUnits=deg
  ArcPx : sm_lib/Body Elements/Solid  InertiaType=CalculateFromGeometry  Mass=1  MassUnits=kg  CenterOfMass=[0 0 0]  CenterOfMassUnits=m  MomentsOfInertia=[1 1 1]  MomentsOfInertiaUnits=kg*m^2  ProductsOfInertia=[0 0 0]  ProductsOfInertiaUnits=kg*m^2  DensityBased=on  Density=rho  DensityUnits=kg/(m^3)  DoExposeReferenceFrame=on  SerializedFrames=<Frames/>  GraphicType=FromGeometry  MarkerShape=Sphere  MarkerSize=10  GraphicVisPropType=SimpleVisualProperties  GraphicDiffuseColor=clr  GraphicSpecularColor=[0.5 0.5 0.5 1.0]  GraphicAmbientColor=[0.15 0.15 0.15 1.0]  GraphicEmissiveColor=[0.0 0.0 0.0 1.0]  GraphicShininess=75  GraphicOpacity=1.0  GeometryShape=GeneralSolidOfRevolution  RectangleSize=[1 1]  RectangleSizeUnits=m  BrickDimensions=[1 1 1]  BrickDimensionUnits=m  CylinderRadius=1  CylinderRadiusUnits=m  CylinderLength=1  CylinderLengthUnits=m  SphereRadius=1  SphereRadiusUnits=m  EllipsoidRadii=[1 1 1]  EllipsoidRadiiUnits=m  ExtrusionCrossSection=[1 1; -1 1; -1 -1; 1 -1]  ExtrusionCrossSectionUnits=m  ExtrusionLength=1  ExtrusionLengthUnits=m  PolygonNumSides=3  PolygonOuterRadius=1  PolygonOuterRadiusUnits=m  ExtGeomFileType=STEP  ExtGeomFileUnits=m  RevolutionCrossSection=[[-1 1 1 -1]*pipe_width/2+rail_curve_rad1;[-1 -1 1 1]*pipe_width/2]'  RevolutionCrossSectionUnits=cm  RevolutionExtent=Custom  RevolutionAngle=curve_ang1  RevolutionAngleUnits=deg
  Transform Angle : sm_lib/Frames and Transforms/Rigid Transform  TranslationMethod=Cartesian  TranslationStandardOffset=0  TranslationLengthUnit=cm  TranslationStandardAxis=+X  TranslationCartesianOffset=[-(1-cosd(curve_ang1))*rail_curve_rad1-0.5*(height_c2-height_c1)/tand(90-curve_ang1) 0 height_c1+sind(curve_ang1)*rail_curve_rad1+(height_c2-height_c1)*0.5]  TranslationROffset=0  TranslationROffsetUnits=m  TranslationZOffset=0  TranslationZOffsetUnits=m  TranslationThetaOffset=0  TranslationThetaOffsetUnits=deg  RotationMethod=StandardAxis  RotationAngleUnits=deg  RotationStandardAxis=-Y  RotationAngle=curve_ang1  RotationArbitraryAxis=[0 0 1]  FollAlignAxisA=+X  BaseAlignAxisA=+Y  FollAlignAxisB=+Y  BaseAlignAxisB=+Z  RotationSequenceAxes=FollowerAxes  RotationSequence=XYX  RotationSequenceAngles=[0 0 0]  RotationSequenceAnglesUnits=deg  RotationMatrix=[1 0 0; 0 1 0; 0 0 1]
  Transform ArcPx : sm_lib/Frames and Transforms/Rigid Transform  TranslationMethod=Cartesian  TranslationStandardOffset=0  TranslationLengthUnit=cm  TranslationStandardAxis=+Z  TranslationCartesianOffset=[-rail_curve_rad1 0 height_c1]  TranslationROffset=0  TranslationROffsetUnits=m  TranslationZOffset=0  TranslationZOffsetUnits=m  TranslationThetaOffset=0  TranslationThetaOffsetUnits=deg  RotationMethod=RotationSequence  RotationAngleUnits=deg  RotationStandardAxis=+X  RotationAngle=90.0  RotationArbitraryAxis=[0 0 1]  FollAlignAxisA=+X  BaseAlignAxisA=+Y  FollAlignAxisB=+Y  BaseAlignAxisB=+Z  RotationSequenceAxes=BaseAxes  RotationSequence=XYX  RotationSequenceAngles=[90 -curve_ang1/2 0]  RotationSequenceAnglesUnits=deg  RotationMatrix=[1 0 0; 0 1 0; 0 0 1]
  Transform Horiz : sm_lib/Frames and Transforms/Rigid Transform  TranslationMethod=Cartesian  TranslationStandardOffset=0  TranslationLengthUnit=cm  TranslationStandardAxis=+Z  TranslationCartesianOffset=[-1*(width+rail_curve_rad1+(height_c2-height_c1)/tand(90-curve_ang1))*0.5-pipe_width/2*0 0 height_c2+rail_curve_rad2]  TranslationROffset=0  TranslationROffsetUnits=m  TranslationZOffset=0  TranslationZOffsetUnits=m  TranslationThetaOffset=0  TranslationThetaOffsetUnits=deg  RotationMethod=StandardAxis  RotationAngleUnits=deg  RotationStandardAxis=+Y  RotationAngle=90.0  RotationArbitraryAxis=[0 0 1]  FollAlignAxisA=+X  BaseAlignAxisA=+Y  FollAlignAxisB=+Y  BaseAlignAxisB=+Z  RotationSequenceAxes=FollowerAxes  RotationSequence=XYX  RotationSequenceAngles=[0 0 0]  RotationSequenceAnglesUnits=deg  RotationMatrix=[1 0 0; 0 1 0; 0 0 1]
  Transform Vert Px : sm_lib/Frames and Transforms/Rigid Transform  TranslationMethod=None  TranslationStandardOffset=0  TranslationLengthUnit=cm  TranslationStandardAxis=+X  TranslationCartesianOffset=[0 0 0]  TranslationROffset=0  TranslationROffsetUnits=m  TranslationZOffset=0  TranslationZOffsetUnits=m  TranslationThetaOffset=0  TranslationThetaOffsetUnits=deg  RotationMethod=None  RotationAngleUnits=deg  RotationStandardAxis=+X  RotationAngle=90.0  RotationArbitraryAxis=[0 0 1]  FollAlignAxisA=+X  BaseAlignAxisA=+Y  FollAlignAxisB=+Y  BaseAlignAxisB=+Z  RotationSequenceAxes=FollowerAxes  RotationSequence=XYX  RotationSequenceAngles=[0 0 0]  RotationSequenceAnglesUnits=deg  RotationMatrix=[1 0 0; 0 1 0; 0 0 1]
  Transform Vert Px1 : sm_lib/Frames and Transforms/Rigid Transform  TranslationMethod=Cartesian  TranslationStandardOffset=0  TranslationLengthUnit=cm  TranslationStandardAxis=+X  TranslationCartesianOffset=[-rail_curve_rad1-(height_c2-height_c1)/tand(90-curve_ang1) 0 height_c2]  TranslationROffset=0  TranslationROffsetUnits=m  TranslationZOffset=0  TranslationZOffsetUnits=m  TranslationThetaOffset=0  TranslationThetaOffsetUnits=deg  RotationMethod=RotationSequence  RotationAngleUnits=deg  RotationStandardAxis=+X  RotationAngle=90.0  RotationArbitraryAxis=[0 0 1]  FollAlignAxisA=+X  BaseAlignAxisA=+Y  FollAlignAxisB=+Y  BaseAlignAxisB=+Z  RotationSequenceAxes=BaseAxes  RotationSequence=XYX  RotationSequenceAngles=[90 -(90+curve_ang1)/2 0]  RotationSequenceAnglesUnits=deg  RotationMatrix=[1 0 0; 0 1 0; 0 0 1]
  Vert Nx : sm_lib/Body Elements/Solid  InertiaType=CalculateFromGeometry  Mass=1  MassUnits=kg  CenterOfMass=[0 0 0]  CenterOfMassUnits=m  MomentsOfInertia=[1 1 1]  MomentsOfInertiaUnits=kg*m^2  ProductsOfInertia=[0 0 0]  ProductsOfInertiaUnits=kg*m^2  DensityBased=on  Density=rho  DensityUnits=kg/(m^3)  DoExposeReferenceFrame=on  SerializedFrames=<Frames/>  GraphicType=FromGeometry  MarkerShape=Sphere  MarkerSize=10  GraphicVisPropType=SimpleVisualProperties  GraphicDiffuseColor=clr  GraphicSpecularColor=[0.5 0.5 0.5 1.0]  GraphicAmbientColor=[0.15 0.15 0.15 1.0]  GraphicEmissiveColor=[0.0 0.0 0.0 1.0]  GraphicShininess=75  GraphicOpacity=1.0  GeometryShape=Brick  RectangleSize=[1 1]  RectangleSizeUnits=m  BrickDimensions=[pipe_width pipe_width (width-rail_curve_rad1-(height_c2-height_c1)/tand(90-curve_ang1))-pipe_width/2*0]  BrickDimensionUnits=cm  CylinderRadius=1  CylinderRadiusUnits=cm  CylinderLength=1  CylinderLengthUnits=cm  SphereRadius=1  SphereRadiusUnits=m  EllipsoidRadii=[1 1 1]  EllipsoidRadiiUnits=m  ExtrusionCrossSection=[1 1; -1 1; -1 -1; 1 -1]  ExtrusionCrossSectionUnits=m  ExtrusionLength=1  ExtrusionLengthUnits=m  PolygonNumSides=3  PolygonOuterRadius=1  PolygonOuterRadiusUnits=m  ExtGeomFileType=STEP  ExtGeomFileUnits=m  RevolutionCrossSection=[1 1; 1 -1; 2 -1; 2 1]  RevolutionCrossSectionUnits=m  RevolutionExtent=Full  RevolutionAngle=180  RevolutionAngleUnits=deg
  Vert Px : sm_lib/Body Elements/Solid  InertiaType=CalculateFromGeometry  Mass=1  MassUnits=kg  CenterOfMass=[0 0 0]  CenterOfMassUnits=m  MomentsOfInertia=[1 1 1]  MomentsOfInertiaUnits=kg*m^2  ProductsOfInertia=[0 0 0]  ProductsOfInertiaUnits=kg*m^2  DensityBased=on  Density=rho  DensityUnits=kg/(m^3)  DoExposeReferenceFrame=off  SerializedFrames=<Frames><Frame><Id>Frame1</Id><Value><Name>Bo</Name><Origin><Source>GeometricFeature</Source><FeatureName>-z surface</FeatureName></Origin><PrimaryAxis><DefinedDirection>+Z</DefinedDirection><Source>ReferenceFrame</Source><SourceDirection>+Z</SourceDirection><FeatureName></FeatureName></PrimaryAxis><SecondaryAxis><DefinedDirection>+X</DefinedDirection><Source>ReferenceFrame</Source><SourceDirection>+X</SourceDirection><FeatureName></FeatureName></SecondaryAxis></Value></Frame></Frames>  GraphicType=FromGeometry  MarkerShape=Sphere  MarkerSize=10  GraphicVisPropType=SimpleVisualProperties  GraphicDiffuseColor=clr  GraphicSpecularColor=[0.5 0.5 0.5 1.0]  GraphicAmbientColor=[0.15 0.15 0.15 1.0]  GraphicEmissiveColor=[0.0 0.0 0.0 1.0]  GraphicShininess=75  GraphicOpacity=1.0  GeometryShape=Brick  RectangleSize=[1 1]  RectangleSizeUnits=m  BrickDimensions=[pipe_width pipe_width height_c1]  BrickDimensionUnits=cm  CylinderRadius=1  CylinderRadiusUnits=cm  CylinderLength=1  CylinderLengthUnits=cm  SphereRadius=1  SphereRadiusUnits=m  EllipsoidRadii=[1 1 1]  EllipsoidRadiiUnits=m  ExtrusionCrossSection=[1 1; -1 1; -1 -1; 1 -1]  ExtrusionCrossSectionUnits=m  ExtrusionLength=1  ExtrusionLengthUnits=m  PolygonNumSides=3  PolygonOuterRadius=1  PolygonOuterRadiusUnits=m  ExtGeomFileType=STEP  ExtGeomFileUnits=m  RevolutionCrossSection=[1 1; 1 -1; 2 -1; 2 1]  RevolutionCrossSectionUnits=m  RevolutionExtent=Full  RevolutionAngle=180  RevolutionAngleUnits=deg
  B : PMIOPort  Port=1  Side=Right
  connections:
  Vert Nx/RConn1 -- Transform Horiz/RConn1
  ArcNx/RConn1 -- Transform Vert Px1/RConn1
  ArcPx/RConn1 -- Transform ArcPx/RConn1
  Transform Horiz/LConn1 -- Transform Vert Px1/LConn1 -- B/RConn1 -- Transform Vert Px/LConn1 -- Transform Angle/LConn1
  Vert Px/LConn1 -- Transform ArcPx/LConn1 -- Transform Vert Px/RConn1
  Angle/RConn1 -- Transform Angle/RConn1
